simulink model "Double_Loop_Controller"  (R2016a)
settings: Solver=VariableStepAuto  StartTime=0.0  StopTime=10  RelTol=1e-3
libraries: fl_lib x23, elec_lib x18, nesl_utility x15, pe_lib x5, simulink x2, powerlib_meascontrol x1
settings Model: Creator=kkfrk  LastModifiedBy=kkfrk

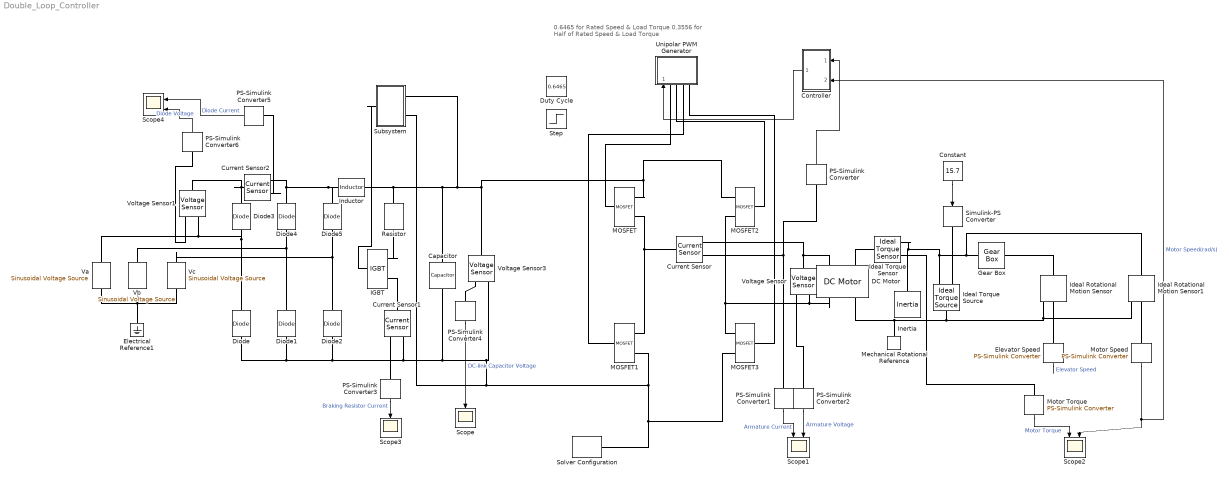
== system Double_Loop_Controller ==
  note: 0.6465 for Rated Speed & Load Torque
      | 0.3556 for Half of Rated Speed & Load Torque
  Capacitor : elec_lib/Passive Devices/Capacitor  enable_table=0  c=1e-3 F  Cvec=[ 1e-5 1e-6 ] F  Vvec=[ 0 10 ] V  CV_table_symmetry=1  C_tol=0.01  enable_C_tol=0  tol_distribution=1  nSigma=4  r=1e-6 Ohm  g=0 1/Ohm  initV=537.8 V  enable_operating_limits=0  operating_limit_action=2  max_working_voltage_range=[ -25 25 ] V  power_rating=1 W  enable_faults=0  fault_action=1  Cscale_faulted=100  R_faulted=0.001 Ohm  G_faulted=0 1/Ohm  tau_fault=0.001 s  enable_temporal_fault=0  t_fault=1 s  enable_behavioral_fault=0  max_permissible_voltage_range=[ -100 100 ] V  t_fail_on_voltage=1 s
  Constant : Constant  Value=15.7
  "Controller " : Subsystem
  Current Sensor : fl_lib/Electrical/Electrical Sensors/Current Sensor
  Current Sensor1 : fl_lib/Electrical/Electrical Sensors/Current Sensor
  Current Sensor2 : fl_lib/Electrical/Electrical Sensors/Current Sensor
  DC Motor : elec_lib/Actuators & Drivers/Rotational Actuators/DC Motor  parameterization=1  Ra=3.68 Ohm  La=32e-3 H  emf_or_torque=1  Kv=1.66 V/(rad/s)  Ki=6.876e-4 N*m/A  T_stall=2.4e-4 N*m  w_max=1.91e+4 rpm  w_rated=1.5e+4 rpm  P_rated=0.08 W  V_rated=1.5 V  J=0.05 kg*m^2  lam_param=1  lam=0 N*m/(rad/s)  i_noload=0 A  V_i_noload=1.5 V  speed0=0 rpm  alpha=0.00393 1/K  Tmeas=25 degC  thermal_mass=100 J/K  initial_temperature=25 degC
  Diode{,1..5} (6 alike) : elec_lib/Semiconductor Devices/Diode  ModelType=1  Vf=0.01 V  Ron=0.01 Ohm  Goff=1e-8 S  Rz=0.3 Ohm  Vz=50 V  C_PWL=5 pF  prmExp=1  I12=[ 0.0137 0.545 ] A  V12=[ 0.6 0.7 ] V  I1=0.0137 A  V1=0.6 V  RS=0.01 Ohm  IS=1e-12 A  Tmeas=25 degC  ec=1  BV=Inf V  C_param=1  CJ0=5 pF  VJ=1 V  Mgrad=0.5  Vvec=[ 0.1 10 100 ] V  Cvec=[ 3.5 1 0.4 ] pF  FC=0.5  Q_param=1  Irrm=-7.15 A  iF=4 A  didt=-750 A/us  trr=115 ns  TT=50 ns  tau=100 ns  T_param=1  IS_T2=1.25e-7 A  I1_T2=0.245 A  V1_T2=0.5 V  Tmeas2=125 degC  EG_param=1  EG=1.11 eV  XTI_param=1  XTI=3  dBVdT=0 V/K  Tdevice=25 degC  Rth=[ 0 10 ] K/W  thermal_mass_parameterization=1  thermal_mass=[ 0 1 ] J/K  thermal_time_constant=[ 0 10 ] s  thermal_mass_initial_temperatures=[ 25 25 ] degC
  Duty Cycle : Constant  Value=0.6465
  Electrical Reference1 : fl_lib/Electrical/Electrical Elements/Electrical Reference
  Elevator Speed : nesl_utility/PS-Simulink Converter  PhysicalDomain=network_engine_domain  SubClassName=ps_output  LeftPortType=input  RightPortType=output  PseudoPeriodic=off  Frequencies=[]  Unit=1  AffineConversion=off
  Gear Box : fl_lib/Mechanical/Mechanisms/Gear Box  ratio=12.5  t_in_specify=off  t_in_priority=None  t_in=0 N*m  t_out_specify=off  t_out_priority=None  t_out=0 N*m
  IGBT : pe_lib/Semiconductors/Fundamental Components/IGBT  Vf=0.8 V  Ron=0.001 Ohm  Goff=1e-5 1/Ohm  Vth=6 V  diode_param=1  diode_Vf=0.8 V  diode_Ron=0.001 Ohm  diode_Goff=1e-5 1/Ohm  diode_C=5e-8 F  diode_iRM=-235 A  diode_iF=300 A  diode_idot=-50 A/us  diode_trr_param=1  diode_trr_factor=3  diode_trr=15 us  diode_Qrr=1.5e+3 s*uA  thermal_loss_option=2  Voff=300 V  Tau=1e-4 s  Tj=[ 298.15 398.15 ] K  Iout_data=[ 0 10 50 100 200 400 600 ] A  Eon_data=[ 0 2.9e-4 0.00143 0.00286 0.00571 0.01314 0.02286; 0 5.7e-4 0.00263 0.00514 0.01029 0.02057 0.03029 ] J  Eoff_data=[ 0 2.1e-4 0.00107 0.00214 0.00429 0.009859999999999999 0.01714; 0 4.3e-4 0.00197 0.00386 0.00771 0.01543 0.02271 ] J  Von_data=[ 0 1.1 1.3 1.45 1.75 2.25 2.7; 0 1 1.15 1.35 1.7 2.35 3 ] V
  Ideal Rotational Motion Sensor : fl_lib/Mechanical/Mechanical Sensors/Ideal Rotational Motion Sensor  offset=0 rad
  Ideal Rotational Motion Sensor1 : fl_lib/Mechanical/Mechanical Sensors/Ideal Rotational Motion Sensor  offset=0 rad
  Ideal Torque Sensor : fl_lib/Mechanical/Mechanical Sensors/Ideal Torque Sensor
  Ideal Torque Source : fl_lib/Mechanical/Mechanical Sources/Ideal Torque Source
  Inductor : elec_lib/Passive Devices/Inductor  l=40e-3 H  L_tol=0.01  enable_L_tol=0  tol_distribution=1  nSigma=4  r=0 Ohm  g=1e-9 1/Ohm  initI=0 A  enable_operating_limits=0  operating_limit_action=2  max_working_current=1 A  power_rating=1 W  enable_faults=0  fault_action=1  lambdaPercent=50  k_faulted=0.9999 Ohm  turnsShort=0  openCct=0  groundShort=0  groundShortG=0 1/Ohm  tau_fault=0.001 s  enable_temporal_fault=0  t_fault=1 s  enable_behavioral_fault=0  max_permissible_voltage=100 V  n_fail_on_voltage=1  max_permissible_current=1 A  t_fail_on_current=1 s
  Inertia : fl_lib/Mechanical/Rotational Elements/Inertia  inertia=0.0512 kg*m^2  w_specify=off  w_priority=High  w=0 rad/s  t_specify=off  t_priority=None  t=0 N*m
  MOSFET{,1..3} (4 alike) : pe_lib/Semiconductors/Fundamental Components/MOSFET  Rds=0.001 Ohm  Goff=1e-6 1/Ohm  Vth=1.1 V  diode_param=2  diode_Vf=0.8 V  diode_Ron=0.001 Ohm  diode_Goff=1e-5 1/Ohm  diode_C=5e-8 F  diode_iRM=-235 A  diode_iF=300 A  diode_idot=-50 A/us  diode_trr_param=1  diode_trr_factor=3  diode_trr=15 us  diode_Qrr=1.5e+3 s*uA
  Mechanical Rotational Reference : fl_lib/Mechanical/Rotational Elements/Mechanical Rotational Reference
  Motor Speed : nesl_utility/PS-Simulink Converter  PhysicalDomain=network_engine_domain  SubClassName=ps_output  LeftPortType=input  RightPortType=output  PseudoPeriodic=off  Frequencies=[]  Unit=1  AffineConversion=off
  Motor Torque : nesl_utility/PS-Simulink Converter  PhysicalDomain=network_engine_domain  SubClassName=ps_output  LeftPortType=input  RightPortType=output  PseudoPeriodic=off  Frequencies=[]  Unit=1  AffineConversion=off
  PS-Simulink Converter{,1..6} (7 alike) : nesl_utility/PS-Simulink Converter  PhysicalDomain=network_engine_domain  SubClassName=ps_output  LeftPortType=input  RightPortType=output  PseudoPeriodic=off  Frequencies=[]  Unit=1  AffineConversion=off
  Resistor : elec_lib/Passive Devices/Resistor  R=13 Ohm  R_tol=5  enable_R_tol=0  tol_distribution=1  nSigma=4  enable_operating_limits=0  operating_limit_action=2  max_working_voltage=100 V  power_rating=1 W  enable_faults=0  fault_action=1  R_faulted=Inf Ohm  enable_temporal_fault=0  t_fault=1 s  enable_behavioral_fault=0  max_permissible_current=1 A  t_fail_on_current=1 s  noise_mode=0  sample_time=0.001 s  repeatability=1  auto_seed=1704206589  user_seed=0  Tdevice=25 degC  alpha=0.00393 1/K  Tmeas=25 degC  thermal_mass=100 J/K  initial_temperature=25 degC  power_derating_T1=70 degC  power_derating_T2=155 degC  operating_temperature_range_vec=[ -50 150 ] degC
  Scope : Scope
  Scope1 : Scope  NumInputPorts=2
  Scope2 : Scope  NumInputPorts=2
  Scope3 : Scope
  Scope4 : Scope  NumInputPorts=2
  Simulink-PS Converter : nesl_utility/Simulink-PS Converter  PhysicalDomain=network_engine_domain  SubClassName=ps_input  LeftPortType=input  RightPortType=output  PseudoPeriodic=off  Frequencies=[]  NoiseDistribution=none  NoiseParameters=[]  Unit=1  AffineConversion=off  InputFiltering=off  SimscapeFilterOrder=1  InputFilterTimeConstant=0.001  UdotUserProvided=1
  Solver Configuration : nesl_utility/Solver Configuration  PhysicalDomain=network_engine_domain  SubClassName=solver  LeftPortType=input  RightPortType=generic  Accelerate=off  Tones=[]  Harmonics=[]  SimulateNoise=off  Profile=off  UseLocalSampling=off  EnableSwitchedLinearOptims=on  FrequencyDomain=off  UseCCode=off  RelTol=0.001  AbsTol=1e-06  MinStep=1e-09  ToWorkspace=off  RevertToSquareIcSolve=off  NumHomotopyIterations=100  PhasorMode=off  PhasorModeNumHarmonics=1  OverrideAbsTol=off  DoDC=off  ResidualTolerance=1e-09  UseLocalSolver=on  LocalSolverChoice=NE_BACKWARD_EULER_ADVANCER  LocalSolverSampleTime=1/60000  DoFixedCost=on  MaxNonlinIter=3  MaxModeIter=2  LinearAlgebra=Sparse  DelaysMemoryBudget=10*4096  AutomaticFiltering=on  FilteringTimeConstant=0.001
  Step : Step  Time=2  Before=0.6465  After=0.3556  SampleTime=0
  Subsystem : Subsystem
  Unipolar PWM Generator : Subsystem
  Va : elec_lib/Additional Components/SPICE-Compatible Components/Sources/Sinusoidal Voltage Source  VO=0 V  VA=230*sqrt(2) V  FREQ=50 Hz  TD=0 ms  DF=0 1/s  OMEGA=0 rad/s
  Vb : elec_lib/Additional Components/SPICE-Compatible Components/Sources/Sinusoidal Voltage Source  VO=0 V  VA=230*sqrt(2) V  FREQ=50 Hz  TD=20/3 ms  DF=0 1/s  OMEGA=0 rad/s
  Vc : elec_lib/Additional Components/SPICE-Compatible Components/Sources/Sinusoidal Voltage Source  VO=0 V  VA=230*sqrt(2) V  FREQ=50 Hz  TD=-20/3 ms  DF=0 1/s  OMEGA=0 rad/s
  Voltage Sensor : fl_lib/Electrical/Electrical Sensors/Voltage Sensor
  Voltage Sensor1 : fl_lib/Electrical/Electrical Sensors/Voltage Sensor
  Voltage Sensor3 : fl_lib/Electrical/Electrical Sensors/Voltage Sensor
  wires:
  Constant/1 -> Simulink-PS Converter/1
  PS-Simulink Converter2/1 -> Scope1/2  "Armature Voltage"
  PS-Simulink Converter1/1 -> Scope1/1  "Armature Current"
  Elevator Speed/1 -> ?  "Elevator Speed"
  Motor Speed/1 -> "Controller "/2(In2), Scope2/2  "Motor Speed(rad/s)"
  Motor Torque/1 -> Scope2/1  "Motor Torque"
  PS-Simulink Converter4/1 -> Scope/1  "DC-link Capacitor Voltage"
  PS-Simulink Converter3/1 -> Scope3/1  "Braking Resistor Current"
  PS-Simulink Converter/1 -> "Controller "/1(In1)
  "Controller "/1(Out1) -> Unipolar PWM Generator/1(In1)
  PS-Simulink Converter5/1 -> Scope4/1  "Diode Current"
  PS-Simulink Converter6/1 -> Scope4/2  "Diode Voltage"
  connections:
  Capacitor/LConn1 -- Subsystem/LConn1 -- MOSFET2/RConn1 -- MOSFET/RConn1 -- Voltage Sensor3/LConn1 -- Resistor/LConn1 -- Inductor/RConn1
  MOSFET/RConn2 -- MOSFET1/RConn1 -- Current Sensor/LConn1
  MOSFET2/RConn2 -- MOSFET3/RConn1 -- Voltage Sensor/RConn2 -- DC Motor/RConn1
  Mechanical Rotational Reference/LConn1 -- Ideal Rotational Motion Sensor1/RConn1 -- Ideal Rotational Motion Sensor/RConn1 -- Ideal Torque Source/LConn1 -- DC Motor/RConn2
  Current Sensor/RConn2 -- DC Motor/LConn1 -- Voltage Sensor/LConn1
  Gear Box/LConn1 -- Ideal Torque Sensor/RConn1 -- Inertia/LConn1 -- Ideal Torque Source/RConn2 -- Ideal Rotational Motion Sensor1/LConn1
  Unipolar PWM Generator/LConn4 -- MOSFET3/LConn1
  Unipolar PWM Generator/LConn2 -- MOSFET2/LConn1
  PS-Simulink Converter1/LConn1 -- PS-Simulink Converter/LConn1 -- Current Sensor/RConn1
  Unipolar PWM Generator/LConn1 -- MOSFET/LConn1
  Ideal Rotational Motion Sensor/LConn1 -- Gear Box/RConn1
  Ideal Torque Sensor/RConn2 -- Motor Torque/LConn1
  Elevator Speed/LConn1 -- Ideal Rotational Motion Sensor/RConn2
  Ideal Rotational Motion Sensor1/RConn2 -- Motor Speed/LConn1
  Simulink-PS Converter/RConn1 -- Ideal Torque Source/RConn1
  PS-Simulink Converter2/LConn1 -- Voltage Sensor/RConn1
  Unipolar PWM Generator/LConn3 -- MOSFET1/LConn1
  Diode1/RConn1 -- Vb/LConn1 -- Diode4/LConn1
  MOSFET3/RConn2 -- Subsystem/LConn2 -- Current Sensor1/RConn2 -- Diode2/LConn1 -- Diode1/LConn1 -- Diode/LConn1 -- Capacitor/RConn1 -- Voltage Sensor3/RConn2 -- MOSFET1/RConn2 -- Solver Configuration/RConn1
  Diode/RConn1 -- Voltage Sensor1/RConn2 -- Va/LConn1 -- Diode3/LConn1
  Inductor/LConn1 -- Current Sensor2/RConn2 -- Diode4/RConn1 -- Diode5/RConn1
  Diode2/RConn1 -- Vc/LConn1 -- Diode5/LConn1
  Vb/RConn1 -- Electrical Reference1/LConn1 -- Va/RConn1 -- Vc/RConn1
  PS-Simulink Converter4/LConn1 -- Voltage Sensor3/RConn1
  IGBT/RConn1 -- Resistor/RConn1
  Subsystem/RConn1 -- IGBT/LConn1
  IGBT/RConn2 -- Current Sensor1/LConn1
  PS-Simulink Converter3/LConn1 -- Current Sensor1/RConn1
  DC Motor/LConn2 -- Ideal Torque Sensor/LConn1
  Current Sensor2/LConn1 -- Diode3/RConn1 -- Voltage Sensor1/LConn1
  Current Sensor2/RConn1 -- PS-Simulink Converter5/LConn1
  Voltage Sensor1/RConn1 -- PS-Simulink Converter6/LConn1

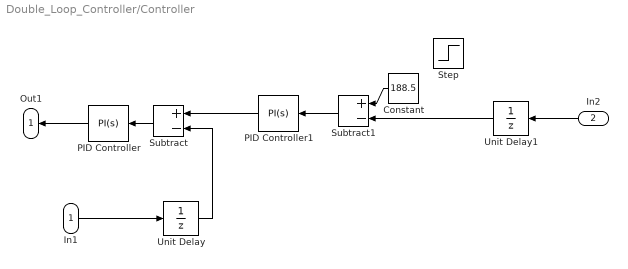
== system Double_Loop_Controller/Controller  ==
  In1 : Inport
  In2 : Inport  Port=2
  Constant : Constant  Value=188.5
  PID Controller : simulink/Continuous/PID Controller  Controller=PI  TimeDomain=Continuous-time  SampleTime=-1  IntegratorMethod=Forward Euler  FilterMethod=Forward Euler  Form=Parallel  UseFilter=on  ControllerParametersSource=internal  P=30  I=0.1  D=0  N=100  InitialConditionSource=internal  InitialConditionForIntegrator=0  InitialConditionForFilter=0  ExternalReset=none  LimitOutput=on  UpperSaturationLimit=1  LowerSaturationLimit=0  LinearizeAsGain=on  AntiWindupMode=none  Kb=1  TrackingMode=off  Kt=1  PParamMin=[]  PParamMax=[]  IParamMin=[]  IParamMax=[]  DParamMin=[]  DParamMax=[]  NParamMin=[]  NParamMax=[]  KbParamMin=[]  KbParamMax=[]  KtParamMin=[]  KtParamMax=[]  POutMin=[]  POutMax=[]  IOutMin=[]  IOutMax=[]  DOutMin=[]  DOutMax=[]  NOutMin=[]  NOutMax=[]  KbOutMin=[]  KbOutMax=[]  KtOutMin=[]  KtOutMax=[]  IntegratorOutMin=[]  IntegratorOutMax=[]  FilterOutMin=[]  FilterOutMax=[]  SumOutMin=[]  SumOutMax=[]  SumI1OutMin=[]  SumI1OutMax=[]  SumI2OutMin=[]  SumI2OutMax=[]  SumI3OutMin=[]  SumI3OutMax=[]  SumDOutMin=[]  SumDOutMax=[]  SaturationOutMin=[]  SaturationOutMax=[]  IntegratorContinuousStateAttributes=''  IntegratorStateMustResolveToSignalObject=off  IntegratorRTWStateStorageClass=Auto  FilterContinuousStateAttributes=''  FilterStateMustResolveToSignalObject=off  FilterRTWStateStorageClass=Auto  DifferentiatorICPrevScaledInput=0  DifferentiatorOutMin=[]  DifferentiatorOutMax=[]
  PID Controller1 : simulink/Continuous/PID Controller  Controller=PI  TimeDomain=Continuous-time  SampleTime=-1  IntegratorMethod=Forward Euler  FilterMethod=Forward Euler  Form=Parallel  UseFilter=on  ControllerParametersSource=internal  P=0.1  I=0.05  D=0.5  N=100  InitialConditionSource=internal  InitialConditionForIntegrator=0  InitialConditionForFilter=0  ExternalReset=none  LimitOutput=off  UpperSaturationLimit=1  LowerSaturationLimit=0  LinearizeAsGain=on  AntiWindupMode=none  Kb=1  TrackingMode=off  Kt=1  PParamMin=[]  PParamMax=[]  IParamMin=[]  IParamMax=[]  DParamMin=[]  DParamMax=[]  NParamMin=[]  NParamMax=[]  KbParamMin=[]  KbParamMax=[]  KtParamMin=[]  KtParamMax=[]  POutMin=[]  POutMax=[]  IOutMin=[]  IOutMax=[]  DOutMin=[]  DOutMax=[]  NOutMin=[]  NOutMax=[]  KbOutMin=[]  KbOutMax=[]  KtOutMin=[]  KtOutMax=[]  IntegratorOutMin=[]  IntegratorOutMax=[]  FilterOutMin=[]  FilterOutMax=[]  SumOutMin=[]  SumOutMax=[]  SumI1OutMin=[]  SumI1OutMax=[]  SumI2OutMin=[]  SumI2OutMax=[]  SumI3OutMin=[]  SumI3OutMax=[]  SumDOutMin=[]  SumDOutMax=[]  SaturationOutMin=[]  SaturationOutMax=[]  IntegratorContinuousStateAttributes=''  IntegratorStateMustResolveToSignalObject=off  IntegratorRTWStateStorageClass=Auto  FilterContinuousStateAttributes=''  FilterStateMustResolveToSignalObject=off  FilterRTWStateStorageClass=Auto  DifferentiatorICPrevScaledInput=0  DifferentiatorOutMin=[]  DifferentiatorOutMax=[]
  Step : Step  Time=10  Before=188.5  After=0  SampleTime=0
  Subtract : Sum  Inputs=+-
  Subtract1 : Sum  Inputs=+-
  Unit Delay : UnitDelay  SampleTime=-1
  Unit Delay1 : UnitDelay  SampleTime=-1
  Out1 : Outport
  wires:
  Unit Delay1/1 -> Subtract1/2
  Subtract1/1 -> PID Controller1/1
  In2/1 -> Unit Delay1/1
  Subtract/1 -> PID Controller/1
  Unit Delay/1 -> Subtract/2
  PID Controller1/1 -> Subtract/1
  In1/1 -> Unit Delay/1
  PID Controller/1 -> Out1/1
  Constant/1 -> Subtract1/1

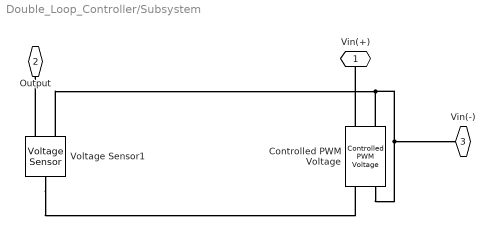
== system Double_Loop_Controller/Subsystem ==
  Controlled PWM Voltage : elec_lib/Actuators & Drivers/Drivers/Controlled PWM Voltage  F=10e3 Hz  TD=0 s  pulse_width_offset=0 s  Vmin=580 V  Vmax=620 V  Vm=10 V  pwm_or_av=1  event_type=1  sample_time=1e-6 s
  Voltage Sensor1 : fl_lib/Electrical/Electrical Sensors/Voltage Sensor
  Vin(+) : PMIOPort  Port=1  Side=Left
  Output : PMIOPort  Port=2  Side=Right
  Vin(-) : PMIOPort  Port=3  Side=Left
  connections:
  Voltage Sensor1/LConn1 -- Controlled PWM Voltage/RConn1
  Controlled PWM Voltage/LConn1 -- Vin(+)/RConn1
  Voltage Sensor1/RConn2 -- Vin(-)/RConn1 -- Controlled PWM Voltage/RConn2 -- Controlled PWM Voltage/LConn2
  Voltage Sensor1/RConn1 -- Output/RConn1

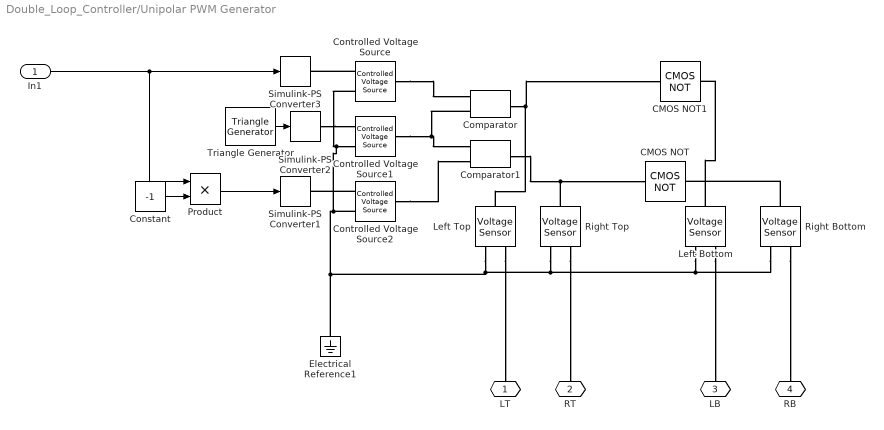
== system Double_Loop_Controller/Unipolar PWM Generator ==
  In1 : Inport
  CMOS NOT : elec_lib/Integrated Circuits/Logic/CMOS NOT  V_IL=1 V  V_IH=10 V  C_IN=5 pF  output_type=1  V_OL=0 V  V_OH=10 V  V_CC=5 V  V_meas=5 V  R_OUT=25 Ohm  R_OH=[ 25 250 ] Ohm  I_OH=63 mA  R_OL=[ 30 800 ] Ohm  I_OL=-45 mA  Delay=25 ns  Ron=5 Ohm  Vf=0.6 V  output_state=1
  CMOS NOT1 : elec_lib/Integrated Circuits/Logic/CMOS NOT  V_IL=1 V  V_IH=10 V  C_IN=5 pF  output_type=1  V_OL=0 V  V_OH=10 V  V_CC=5 V  V_meas=5 V  R_OUT=25 Ohm  R_OH=[ 25 250 ] Ohm  I_OH=63 mA  R_OL=[ 30 800 ] Ohm  I_OL=-45 mA  Delay=25 ns  Ron=5 Ohm  Vf=0.6 V  output_state=1
  Comparator : elec_lib/Integrated Circuits/Comparator  V_OS=1 mV  V_OL=1 V  V_OH=10 V  C_IN=0 pF  R_OUT=50 Ohm  Delay=0 s
  Comparator1 : elec_lib/Integrated Circuits/Comparator  V_OS=1 mV  V_OL=1 V  V_OH=10 V  C_IN=0 pF  R_OUT=50 Ohm  Delay=0 s
  Constant : Constant  Value=-1
  Controlled Voltage Source : fl_lib/Electrical/Electrical Sources/Controlled Voltage Source
  Controlled Voltage Source1 : fl_lib/Electrical/Electrical Sources/Controlled Voltage Source
  Controlled Voltage Source2 : fl_lib/Electrical/Electrical Sources/Controlled Voltage Source
  Electrical Reference1 : fl_lib/Electrical/Electrical Elements/Electrical Reference
  Left Bottom : fl_lib/Electrical/Electrical Sensors/Voltage Sensor
  Left Top : fl_lib/Electrical/Electrical Sensors/Voltage Sensor
  Product : Product
  Right Bottom : fl_lib/Electrical/Electrical Sensors/Voltage Sensor
  Right Top : fl_lib/Electrical/Electrical Sensors/Voltage Sensor
  Simulink-PS Converter1 : nesl_utility/Simulink-PS Converter  PhysicalDomain=network_engine_domain  SubClassName=ps_input  LeftPortType=input  RightPortType=output  PseudoPeriodic=off  Frequencies=[]  NoiseDistribution=none  NoiseParameters=[]  Unit=1  AffineConversion=off  InputFiltering=off  SimscapeFilterOrder=1  InputFilterTimeConstant=0.001  UdotUserProvided=1
  Simulink-PS Converter2 : nesl_utility/Simulink-PS Converter  PhysicalDomain=network_engine_domain  SubClassName=ps_input  LeftPortType=input  RightPortType=output  PseudoPeriodic=off  Frequencies=[]  NoiseDistribution=none  NoiseParameters=[]  Unit=1  AffineConversion=off  InputFiltering=off  SimscapeFilterOrder=1  InputFilterTimeConstant=0.001  UdotUserProvided=1
  Simulink-PS Converter3 : nesl_utility/Simulink-PS Converter  PhysicalDomain=network_engine_domain  SubClassName=ps_input  LeftPortType=input  RightPortType=output  PseudoPeriodic=off  Frequencies=[]  NoiseDistribution=none  NoiseParameters=[]  Unit=1  AffineConversion=off  InputFiltering=off  SimscapeFilterOrder=1  InputFilterTimeConstant=0.001  UdotUserProvided=1
  Triangle Generator : powerlib_meascontrol/Pulse & Signal Generators/Triangle Generator  Freq=15e3  Phase=90  Ts=0
  LT : PMIOPort  Port=1  Side=Left
  RT : PMIOPort  Port=2  Side=Left
  LB : PMIOPort  Port=3  Side=Left
  RB : PMIOPort  Port=4  Side=Left
  wires:
  In1/1 -> Product/1, Simulink-PS Converter3/1
  Triangle Generator/1 -> Simulink-PS Converter2/1
  Product/1 -> Simulink-PS Converter1/1
  Constant/1 -> Product/2
  connections:
  Controlled Voltage Source/RConn2 -- Right Bottom/RConn2 -- Left Bottom/RConn2 -- Right Top/RConn2 -- Left Top/RConn2 -- Electrical Reference1/LConn1 -- Controlled Voltage Source2/RConn2 -- Controlled Voltage Source1/RConn2
  Left Bottom/LConn1 -- CMOS NOT1/RConn1
  Controlled Voltage Source2/LConn1 -- Comparator1/LConn1
  Left Bottom/RConn1 -- LB/RConn1
  Comparator/RConn1 -- Left Top/LConn1 -- CMOS NOT1/LConn1
  Controlled Voltage Source/RConn1 -- Simulink-PS Converter3/RConn1
  Left Top/RConn1 -- LT/RConn1
  Right Top/RConn1 -- RT/RConn1
  Right Bottom/RConn1 -- RB/RConn1
  Controlled Voltage Source/LConn1 -- Comparator/LConn1
  Controlled Voltage Source2/RConn1 -- Simulink-PS Converter1/RConn1
  Controlled Voltage Source1/LConn1 -- Comparator/LConn2 -- Comparator1/LConn2
  Simulink-PS Converter2/RConn1 -- Controlled Voltage Source1/RConn1
  Comparator1/RConn1 -- Right Top/LConn1 -- CMOS NOT/LConn1
  Right Bottom/LConn1 -- CMOS NOT/RConn1
